simulink model "RM3_FLC"  (R2015b)
settings: Solver=ode4  StartTime=0  StopTime=200  FixedStep=0.01  MaxStep=0.01  RelTol=1e-3
values from neighbouring files (symbols this model uses):
  simu = simulationClass()    [wecSimInputFile.m]
  waves = waveClass('irregular')    [wecSimInputFile.m]
undefined symbols (not defined in the file or in its folder): body, constraint, pto
libraries: WECSim_Lib x5
settings Model: Creator=mlawson  LastModifiedBy=dforbus
settings SolverCC: ZeroCrossControl=DisableAll  AlgebraicLoopSolver=LineSearch  AutoInsertRateTranBlk=on
settings DataIOCC: LimitDataPoints=off  SaveFormat=Array  SaveOutput=off  SaveTime=off
settings OptimizationCC: SimCompilerOptimization=on
settings DebuggingCC: UnderspecifiedInitializationDetection=Classic  MergeDetectMultiDrivingBlocksExec=none  SolverPrmCheckMsg=warning  StateNameClashWarn=warning
settings HardwareCC: ProdBitPerPointer=32  ProdLargestAtomicFloat=None  ProdIntDivRoundTo=Undefined  ProdEndianess=Unspecified  ProdWordSize=32  ProdHWDeviceType=32-bit Generic
settings GRTTargetCC: GeneratePreprocessorConditionals=Disable all
settings ConfigComp: CovModelRefEnable=Off  CovSFcnEnable=off
settings SimscapeCC: SimscapeNormalizeSystem=off
settings ExplorerConfigSet: InternalSimMechanicsExplorerSettings="<ExplorerConfiguration><canonicalview>default</canonicalview><TilePanel><TileInfo><Tiles Columns=\"1\" Count=\"1\" Rows=\"1\"><Column Left=\"2\" Weight=\"1\"/><Column Left=\"1335\"/><Row Top=\"2\" Weight=\"1\"/><Row Top=\"911\"/><Tile Height=\"1\" Width=\"1\" X=\"0\" Y=\"0\"/></Tiles></TileInfo><SceneInfo><SceneViewer><BGColor><R>0.60000002384185791</R><G>0.60000002384185791</G><B>0.60000002384185791</B></BGColor><Camera><Position><X>365.37645888990272</X><Y>-369.82486814446582</Y><Z>359.64809521743916</Z></Position><Center><X>-6.7351450971904585</X><Y>2.2867358426280204</Y><Z>-12.463508769654169</Z></Center><Up><X>-0.40824829046386307</X><Y>0.40824829046386307</Y><Z>0.81649658092772615</Z></Up><Left>-57.820127362122818</Left><Right>57.820127362122818</Right><Bottom>-38.308817187253304</Bottom><Top>38.308817187253304</Top></Camera></SceneViewer></SceneInfo></TilePanel></ExplorerConfiguration>"

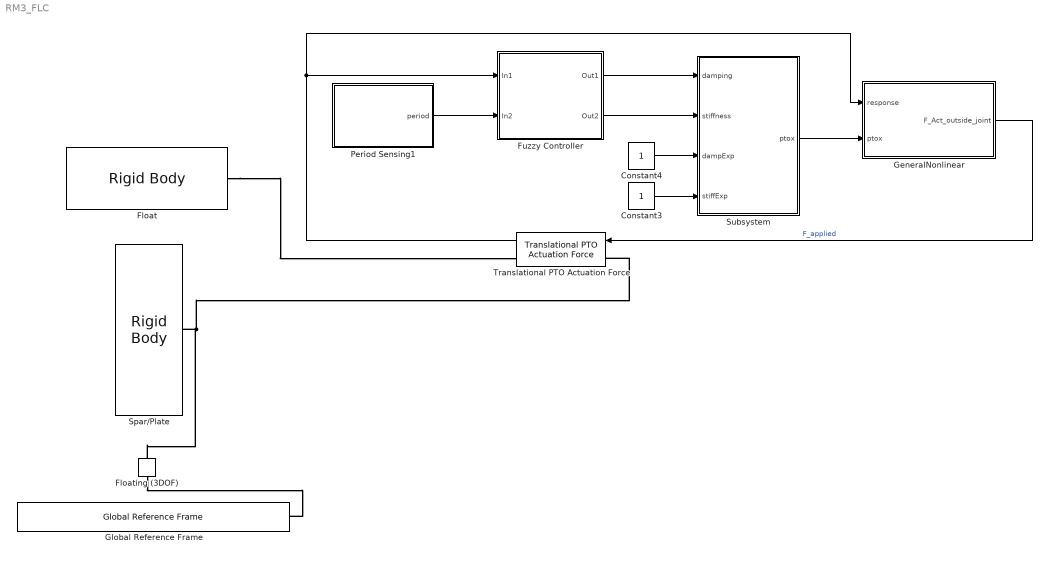
== system RM3_FLC ==
  Constant3 : Constant
  Constant4 : Constant
  Float : WECSim_Lib/Body Elements/Rigid Body  body=body(1)
      settings: AttributesFormatString=%<body>
  Floating (3DOF) : WECSim_Lib/Constraints/Floating (3DOF)  constraint=constraint(1)
      settings: AttributesFormatString=%<constraint>
  Fuzzy Controller : Subsystem
  GeneralNonlinear : Subsystem
  Global Reference Frame : WECSim_Lib/Frames/Global Reference Frame  waves=waves  simu=simu
  Period Sensing1 : Subsystem
  Spar/Plate : WECSim_Lib/Body Elements/Rigid Body  body=body(2)
      settings: AttributesFormatString=%<body>
  Subsystem : Subsystem
  Translational PTO Actuation Force : WECSim_Lib/PTOs/Translational PTO Actuation Force  pto=pto(1)
      settings: AttributesFormatString=%<pto>
  wires:
  Constant3/1 -> Subsystem/4(stiffExp)
  Subsystem/1(ptox) -> GeneralNonlinear/2(ptox)
  GeneralNonlinear/1(F_Act_outside_joint) -> Translational PTO Actuation Force/1  "F_applied"
  Constant4/1 -> Subsystem/3(dampExp)
  Translational PTO Actuation Force/1 -> GeneralNonlinear/1(response), Fuzzy Controller/1(In1)
  Fuzzy Controller/2(Out2) -> Subsystem/2(stiffness)
  Fuzzy Controller/1(Out1) -> Subsystem/1(damping)
  Period Sensing1/1(period) -> Fuzzy Controller/2(In2)
  connections:
  Floating (3DOF)/LConn1 -- Global Reference Frame/RConn1
  Spar/Plate/RConn1 -- Translational PTO Actuation Force/LConn1 -- Floating (3DOF)/RConn1
  Float/RConn1 -- Translational PTO Actuation Force/RConn1

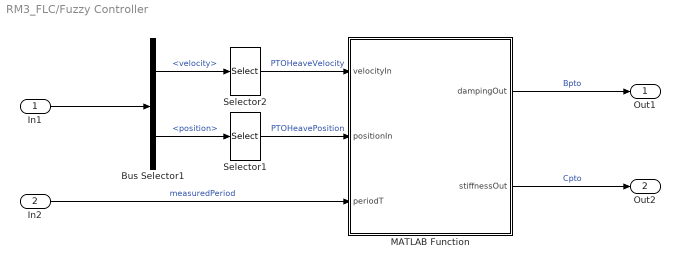
== system RM3_FLC/Fuzzy Controller ==
  In1 : Inport
  In2 : Inport  Port=2
  Bus Selector1 : BusSelector  OutputSignals=velocity,position
  MATLAB Function : MATLAB Function  TreatAsAtomicUnit=on  SystemSampleTime=0.01
  Selector1 : Selector  InputPortWidth=6  IndexOptions=Index vector (dialog)  Indices=3  OutputSizes=1
  Selector2 : Selector  InputPortWidth=6  IndexOptions=Index vector (dialog)  Indices=3  OutputSizes=1
  Out1 : Outport
  Out2 : Outport  Port=2
  wires:
  Bus Selector1/2 -> Selector1/1  "<position>"
  Selector2/1 -> MATLAB Function/1(velocityIn)  "PTOHeaveVelocity"
  Bus Selector1/1 -> Selector2/1  "<velocity>"
  In1/1 -> Bus Selector1/1
  Selector1/1 -> MATLAB Function/2(positionIn)  "PTOHeavePosition"
  MATLAB Function/1(dampingOut) -> Out1/1  "Bpto"
  MATLAB Function/2(stiffnessOut) -> Out2/1  "Cpto"
  In2/1 -> MATLAB Function/3(periodT)  "measuredPeriod"

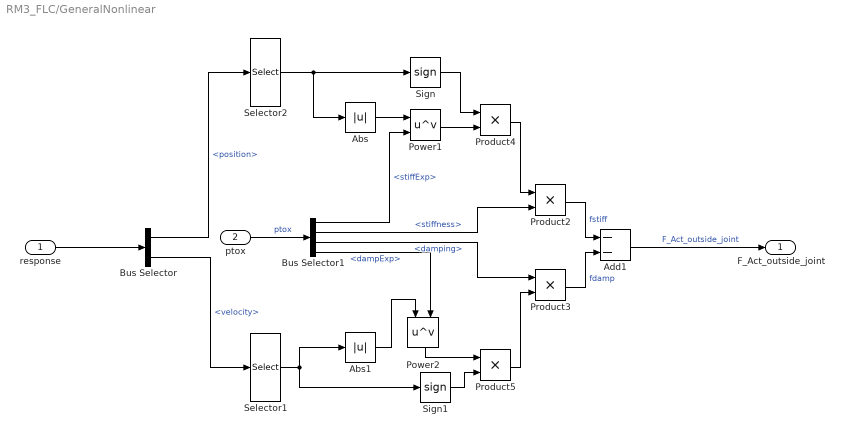
== system RM3_FLC/GeneralNonlinear ==
  response : Inport
  ptox : Inport  Port=2
  Abs : Abs
  Abs1 : Abs
  Add1 : Sum  Inputs=--
  Bus Selector : BusSelector  OutputSignals=position,velocity
  Bus Selector1 : BusSelector  OutputSignals=stiffExp,stiffness,damping,dampExp
  Power1 : Math  Operator=pow  SaturateOnIntegerOverflow=on
  Power2 : Math  Operator=pow  SaturateOnIntegerOverflow=on
  Product2 : Product  Inputs=**
  Product3 : Product  Inputs=**
  Product4 : Product
  Product5 : Product
  Selector1 : Selector  InputPortWidth=6  IndexOptions=Index vector (dialog)  Indices=3  OutputSizes=1
  Selector2 : Selector  InputPortWidth=6  IndexOptions=Index vector (dialog)  Indices=3  OutputSizes=1
  Sign : Signum
  Sign1 : Signum
  F_Act_outside_joint : Outport
  wires:
  Power2/1 -> Product5/1
  Product5/1 -> Product3/2
  Sign/1 -> Product4/1
  Bus Selector1/3 -> Product3/1  "<damping>"
  Product2/1 -> Add1/1  "fstiff"
  response/1 -> Bus Selector/1
  Bus Selector1/1 -> Power1/2  "<stiffExp>"
  Bus Selector/2 -> Selector1/1  "<velocity>"
  Selector2/1 -> Sign/1, Abs/1
  Product4/1 -> Product2/1
  Add1/1 -> F_Act_outside_joint/1  "F_Act_outside_joint"
  Abs1/1 -> Power2/1
  Product3/1 -> Add1/2  "fdamp"
  Sign1/1 -> Product5/2
  Bus Selector1/2 -> Product2/2  "<stiffness>"
  Selector1/1 -> Abs1/1, Sign1/1
  Power1/1 -> Product4/2
  Bus Selector/1 -> Selector2/1  "<position>"
  Abs/1 -> Power1/1
  ptox/1 -> Bus Selector1/1  "ptox"
  Bus Selector1/4 -> Power2/2  "<dampExp>"

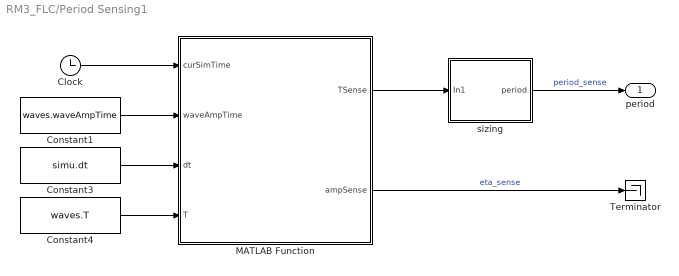
== system RM3_FLC/Period Sensing1 ==
  Clock : Clock
  Constant1 : Constant  Value=waves.waveAmpTime
  Constant3 : Constant  Value=simu.dt
  Constant4 : Constant  Value=waves.T
  MATLAB Function : MATLAB Function  TreatAsAtomicUnit=on  SystemSampleTime=0.1
  Terminator : Terminator
  sizing : Subsystem
  period : Outport
  wires:
  Constant3/1 -> MATLAB Function/3(dt)
  Constant4/1 -> MATLAB Function/4(T)
  MATLAB Function/2(ampSense) -> Terminator/1  "eta_sense"
  sizing/1(period) -> period/1  "period_sense"
  MATLAB Function/1(TSense) -> sizing/1(In1)
  Constant1/1 -> MATLAB Function/2(waveAmpTime)
  Clock/1 -> MATLAB Function/1(curSimTime)

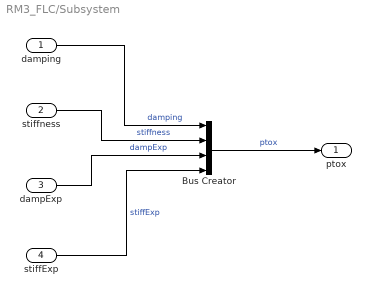
== system RM3_FLC/Subsystem ==
  damping : Inport
  stiffness : Inport  Port=2
  dampExp : Inport  Port=3
  stiffExp : Inport  Port=4
  Bus Creator : BusCreator  Inputs=4
  ptox : Outport
  wires:
  stiffness/1 -> Bus Creator/2  "stiffness"
  stiffExp/1 -> Bus Creator/4  "stiffExp"
  Bus Creator/1 -> ptox/1  "ptox"
  damping/1 -> Bus Creator/1  "damping"
  dampExp/1 -> Bus Creator/3  "dampExp"

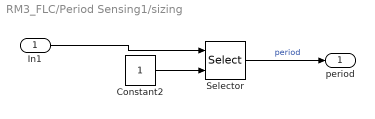
== system RM3_FLC/Period Sensing1/sizing ==
  In1 : Inport
  Constant2 : Constant
  Selector : Selector  InputPortWidth=2  IndexOptions=Index vector (port)  Indices=1  OutputSizes=1
  period : Outport
  wires:
  Constant2/1 -> Selector/2
  In1/1 -> Selector/1
  Selector/1 -> period/1  "period"

== matlab function RM3_FLC/Fuzzy Controller/MATLAB Function ==
  data: velocityIn input; positionIn input; dampingOut output; periodT input; stiffnessOut output
function [dampingOut,stiffnessOut] =...
    fuzzyLogicController(velocityIn, positionIn, periodT)
% Function to create and evaluate a fuzzy logic controller
% which implements a protection system for RM3 to limit relative movement
% between the float and spar, shedding power in the event of too-high wave conditions. The
% PTO implements an optimally linear damped control when within the travel limits,
% and applies a multiplication factor to the damping if the float is close
% to traveling out of bounds

% The functions and structures here are intended to be used as tools for the 
% general application of fuzzy logic controllers to wave energy converters.
% While not as complete as the MATLAB Fuzzy Logic Toolbox, this open source
% framework can be adapted to systems with an arbitrary number of inputs,
% outputs and rules, and can easily be expanded to include more membership
% function types, Fuzzy Operators, implication and aggregation methods, and
% defuzzification rules.

%%%%%%%%%%%%%%%%%%%%%%%%%%%%%%%%%%%%%%%%%%%%%
%% Define input membership functions (MFs) %%
%%%%%%%%%%%%%%%%%%%%%%%%%%%%%%%%%%%%%%%%%%%%%
% Input membership function (MF) structures have the following expected fields:
% type - membership function type. The following linear membership types
%           are defined 'down step' 'step' 'triangle' 'trap'
% definingPoints - the value of the input of the x axis which the linear MF
%           begins changing value e.g. a triangle starts at 0, begins climbing at the
%           first point, peaks at the second, and returns to 0 at the final.
% percentTrue - field to be occupied by the resulting value when the
%            membership function is evaluated at the system input

%%% Period Input %%%
% Min Period
period.MFs.min.type = 'down step';
begin = 3.52; finish = 5.94;
period.MFs.min.definingPoints = [begin finish];
period.MFs.min.percentTrue = NaN;

% Q1 Period
period.MFs.q1.type = 'triangle';
begin = 3.52; peak = 5.94; finish = 6.81;
period.MFs.q1.definingPoints = [begin peak finish];
period.MFs.q1.percentTrue = NaN;

% Med Period
period.MFs.med.type = 'triangle';
begin = 5.94; peak = 6.81; finish = 7.89;
period.MFs.med.definingPoints = [begin peak finish];
period.MFs.med.percentTrue = NaN;

% Q3 Period
period.MFs.q3.type = 'triangle';
begin = 6.81; peak = 7.89; finish = 12.97;
period.MFs.q3.definingPoints = [begin peak finish];
period.MFs.q3.percentTrue = NaN;

% Max Period
period.MFs.max.type = 'step';
begin = 7.89; finish = 12.97;
period.MFs.max.definingPoints = [begin finish];
period.MFs.max.percentTrue = NaN;

%%% Velocity Input %%%
% Too fast Negative Velocity Limit
velocity.MFs.fastNeg.type = 'down step';
begin = -0.50; finish = 0;
velocity.MFs.fastNeg.definingPoints = [begin finish];
velocity.MFs.fastNeg.percentTrue = NaN;

% Too Fast Positive Velocity
velocity.MFs.fastPos.type = 'step';
begin = 0; finish = 0.50;
velocity.MFs.fastPos.definingPoints = [begin finish];
velocity.MFs.fastPos.percentTrue = NaN;

%%% Position Input %%%
% Too Negative Position Limit
position.MFs.low.type = 'down step';
begin = -0.5; finish = -0.4;
position.MFs.low.definingPoints = [begin finish];
position.MFs.low.percentTrue = NaN;

% In spec position
position.MFs.middle.type = 'trap';
begin = -0.5; asc = -0.4; dec = 0.4; finish = 0.5;
position.MFs.middle.definingPoints = [begin asc dec finish];
position.MFs.middle.percentTrue = NaN;

% Too Positive Position
position.MFs.high.type = 'step';
begin = 0.4; finish = 0.5;
position.MFs.high.definingPoints = [begin finish];
position.MFs.high.percentTrue = NaN;

%%%%%%%%%%%%%%%%%%%%
%% Fuzzify Inputs %%
%%%%%%%%%%%%%%%%%%%%
% pass input values to membership functions and update struct with
% membership truth values
period.MFs = fuzzifyInputs(periodT, period.MFs);
position.MFs = fuzzifyInputs(positionIn, position.MFs);
velocity.MFs = fuzzifyInputs(velocityIn, velocity.MFs);


% organize all inputs into a single structure
inputs.period = period;
inputs.position = position;
inputs.velocity = velocity;


%%%%%%%%%%%%%%%%%%%%%%%%%%%
%% Apply Fuzzy Operators %%
%%%%%%%%%%%%%%%%%%%%%%%%%%%
% Define Rule antecedents and apply fuzzy operators to multi-input rules
% Antecedant consist of a vector of the truth values of the applicable membership 
% functions to the rule

% Rule 1 antecedent: If Period is Min
% Single input rule does not require fuzzy operator
ruleOneInputMF = [period.MFs.min.percentTrue];
ruleOneAntecedent = ruleOneInputMF;
ruleSixAntecedent = ruleOneAntecedent; % input set shared with stiffness rule 6

% Rule 2 antecedent: If Period is Q1
% Single input rule does not require fuzzy operator
ruleTwoInputMF = [period.MFs.q1.percentTrue];
ruleTwoAntecedent = ruleTwoInputMF;


% Rule 3 antecedent: If Period is median
% Single input rule does not require fuzzy operator
ruleThreeInputMF = [period.MFs.med.percentTrue];
ruleThreeAntecedent = ruleThreeInputMF;


% Rule 4 antecedent: If Period is Q3
% Single input rule does not require fuzzy operator
ruleFourInputMF = [period.MFs.q3.percentTrue];
ruleFourAntecedent = ruleFourInputMF;


% Rule 5 antecedent: If Period is Max
% Single input rule does not require fuzzy operator
ruleFiveInputMF = [period.MFs.max.percentTrue];
ruleFiveAntecedent = ruleFiveInputMF;
ruleEightAntecedent = ruleFiveAntecedent; % input set shared with stiffness rule 10

% Rule 7 antecedent: If period is q1 or med or q3
ruleSevenInputMFs = [period.MFs.q1.percentTrue period.MFs.med.percentTrue period.MFs.q3.percentTrue];
ruleSevenAntecedent = applyFuzzyOperator(ruleSevenInputMFs, 'sumOr');

% Rule 9 antecedent: If position is middle
% Single input rule does not require fuzzy operator
ruleNineInputMF = [position.MFs.middle.percentTrue];
ruleNineAntecedent = ruleNineInputMF;

% Rule 10 antecedent: If velocity is fast positive and position is high
ruleTenInputMFs = [inputs.velocity.MFs.fastPos.percentTrue  inputs.position.MFs.high.percentTrue];
ruleTenAntecedent = applyFuzzyOperator(ruleTenInputMFs, 'minAnd');

% Rule 11 antecedent: If velocity is fast negative and position is low
ruleElevenInputMFs = [inputs.velocity.MFs.fastNeg.percentTrue  position.MFs.low.percentTrue];
ruleElevenAntecedent = applyFuzzyOperator(ruleElevenInputMFs, 'minAnd');

%%%%%%%%%%%%%%%%%%%%%%%%%%%%
%% Apply Rule Implication %%
%%%%%%%%%%%%%%%%%%%%%%%%%%%%
% Specify membership functions for outputs and Generate Consequent
% Membership Functions (CMFs)

%%% Rules setting PTO Damping (Bpto) %%%

% Rule 1:  If period is min, damping is minDamping
% Base Membership Function
minPdDamping.type = 'impulse';
peak = 258893.62;
minPdDamping.definingPoints = [peak];

% Rule 2:  If period is q1, damping is q1Damping
% Base Membership Function
q1PdDamping.type = 'impulse';
peak = 858598.80;
q1PdDamping.definingPoints = [peak];

% Rule 3:  If period is med, damping is medDamping
% Base Membership Function
medPdDamping.type = 'impulse';
peak = 1353852.40;
medPdDamping.definingPoints = [peak];

% Rule 4:  If period is q3, damping is q3Damping
% Base Membership Function
q3dPdDamping.type = 'impulse';
peak = 2216704.03;
q3PdDamping.definingPoints =[peak];

% Rule 5:  If period is max, damping is maxDamping
% Base Membership Function
maxPdDamping.type = 'impulse';
peak = 35283681.68;
maxPdDamping.definingPoints = [peak];

%%% Rules setting PTO Stiffness (Cpto) %%%
%%% referred to quartiles are for the period, not the Cpto value

% Rule 6:  If period is min, Cpto is minPdStiffness
% Base Membership Function
minPdStiffness.type = 'impulse';
peak = 2480994.89;
minPdStiffness.definingPoints = [peak];

% Rule 7:  If period is q1 or med or q3, Cpto is limitStiffness
% Base Membership Function
limitStiffness.type = 'impulse';
peak = -226644.01;
limitStiffness.definingPoints = [peak];

% Rule 8: If period is max, Cpto is maxPd Stiffness
% Base Membership Function
maxPdStiffness.type = 'impulse';
peak = 14168810.64;
maxPdStiffness.definingPoints = [peak];

% Rule 9:  If position is middle damping is optimal
% Base Membership Function
optimal.type = 'triangle';
begin = -38; peak = 1; finish = 40;
optimal.definingPoints = [begin peak finish];

%%% Rules for position limiting

% Rule 10: If velocity is fast positive and position is high damping is
% overdamped

% Rule 11: If velocity is fast negative and position is low damping is
% overdamped

% Overdamped Membership Function for multiplier
overDamped.type = 'triangle';
begin = 1; peak = 40; finish = 79;
overDamped.definingPoints = [begin peak finish];

% Consequent Membership Functions for Impulse, just multiply by antecedent

% Damping
ruleOne = ruleOneAntecedent*minPdDamping.definingPoints;
ruleTwo = ruleTwoAntecedent*q1PdDamping.definingPoints;
ruleThree = ruleThreeAntecedent*medPdDamping.definingPoints;
ruleFour = ruleFourAntecedent*q3PdDamping.definingPoints;
ruleFive = ruleFiveAntecedent*maxPdDamping.definingPoints;

% Stiffness
ruleSix = ruleSixAntecedent*minPdStiffness.definingPoints;
ruleSeven = ruleSevenAntecedent*limitStiffness.definingPoints;
ruleEight = ruleEightAntecedent*maxPdStiffness.definingPoints;

%Protection
ruleNine = applyImplicationMethod(ruleNineAntecedent,optimal,'min');
ruleTen = applyImplicationMethod(ruleTenAntecedent,overDamped,'min');
ruleEleven = applyImplicationMethod(ruleElevenAntecedent,overDamped,'min');

% organize by: outputs -> fuzzy sets -> rules
% Each output struct expects a CMF field containing the fuzzy sets which
% belong to that output and a range field containing the limits of the
% output
% Each output fuzzy set struct expects a aggregation type for rules which apply
% and a rules struct containing the modified MF for those rules which apply

damping.range = [258893.62 35283681.68];

stiffness.range = [-226644.01 14168810.64];

dampingMultiplier.baseMFs.overDamped = overDamped;
dampingMultiplier.CMFs.overDamped.ruleAggregation = 'max';
dampingMultiplier.CMFs.overDamped.rules.ruleTen = ruleTen;
dampingMultiplier.CMFs.overDamped.rules.ruleEleven = ruleEleven;

dampingMultiplier.baseMFs.optimal = optimal;
dampingMultiplier.CMFs.optimal.rules.ruleNine = ruleNine;

% use NaN for no limit
dampingMultiplier.range = [1 40];

%%%%%%%%%%%%%%%%%%%%%
%% Aggregate Rules %%
%%%%%%%%%%%%%%%%%%%%%
% expected aggregation methods - 

dampRuleValues = ruleOne + ruleTwo + ruleThree + ruleFour + ruleFive;
dampTotalFirings = ruleOneAntecedent + ruleTwoAntecedent + ruleThreeAntecedent + ruleFourAntecedent + ruleFiveAntecedent;

dampingOutRaw = dampRuleValues/dampTotalFirings;


stiffRuleValues = ruleSix + ruleSeven + ruleEight;
stiffTotalFirings = ruleSixAntecedent + ruleSevenAntecedent + ruleEightAntecedent;

stiffnessOut = stiffRuleValues/stiffTotalFirings;

outputs.dampingMultiplier = dampingMultiplier;
outputs.dampingMultiplier.aggregatedFunction = aggregateCMFs(dampingMultiplier, 'max');

%%%%%%%%%%%%%%%%%%%%%%%%%%
%% Defuzzify output MFs %%
%%%%%%%%%%%%%%%%%%%%%%%%%%
% Defuzzify final output membership functions and assign crisp values
% expected defuzzification methods: centroid, bisector, mean of maxima (MOM),
% largest of maxima (LOM), smallest of maxima (SOM)

 if ~(ruleNineAntecedent) && ~(ruleTenAntecedent) && ~(ruleElevenAntecedent)
    dampingFactor = 1; %default if no rules fires
 else
    dampingFactor = defuzzify(outputs.dampingMultiplier, 'bisector');
    if dampingFactor > 1
        dampingFactor = 1; % overdamp only
    end
 end
 
 dampingOutIntermediate = dampingOutRaw*dampingFactor;
 
 dampingOut = dampingOutIntermediate(1);

end
%%%%%%%%%%%%%%%%%%
%% End of Main %%
%%%%%%%%%%%%%%%%%%
% begin supporting functions

function fuzzufiedInput = fuzzifyInputs(inValue, MFs)
% Function to fuzzify crisp input variables
% inputs: 
%   invalue - crisp input value
%   MFs - struct of fuzzy set membership functions for an input
% outputs: 
%   fuzzufiedInput - updated MFs struct with fuzzy truth value for each MF

    % list of memberships for this input
    listMFs = fieldnames(MFs);

    % go through each membership function
    for k=1:numel(listMFs)
        thisMF = MFs.(listMFs{k});

        mfType = thisMF.type;

        %calculate its percentTrue strength based on type
        switch mfType
            case 'triangle'
                MFs.(listMFs{k}).percentTrue = tri_MF(inValue,...
                    MFs.(listMFs{k}).definingPoints(1), MFs.(listMFs{k}).definingPoints(2), MFs.(listMFs{k}).definingPoints(3), 1);
            case 'step'
                MFs.(listMFs{k}).percentTrue = open_trap_right(inValue,...
                     MFs.(listMFs{k}).definingPoints(1), MFs.(listMFs{k}).definingPoints(2), 1);
            case 'down step'
                 MFs.(listMFs{k}).percentTrue = open_trap_left(inValue,...
                     MFs.(listMFs{k}).definingPoints(1), MFs.(listMFs{k}).definingPoints(2), 1);
            case 'trap'
                 MFs.(listMFs{k}).percentTrue = trap(inValue,...
                     MFs.(listMFs{k}).definingPoints(1), MFs.(listMFs{k}).definingPoints(2), MFs.(listMFs{k}).definingPoints(3), MFs.(listMFs{k}).definingPoints(4), 1);
            otherwise
                disp('membership function type not defined');
        end
    end

    fuzzufiedInput = MFs;

end

function membership = tri_MF(inValue, begin, peak, finish, maxTruth)
% Evaluate input according to triangular MF
% inputs: 
%   inValue - system input value 
%   begin - input value triangle begins to rise, before which truth value is 0
%   peak - input value triangle peaks and begins to fall
%   finish - input value triangle returns to 0, after which which truth value is 0
%   maxTruth - truth value for peak input, default 1 for input MFs
% outputs:
%   membership - truth value between 0 and 1 corresponding to the input    
%
    if inValue < peak
        if inValue <= begin
            membership = 0;
        else
            membership = (maxTruth/(peak - begin)) * (inValue-peak) + maxTruth;
        end
    elseif inValue > peak
        if inValue >= finish
            membership = 0;
        else
            membership = ((-1*maxTruth)/(finish - peak)) * (inValue-peak) + maxTruth;
        end
    else
        membership = maxTruth;
    end
end

function membership = open_trap_left(inValue, begin, finish, maxTruth)
% Evaluate input according to falling step membership function
% inputs: 
%   inValue - system input value 
%   begin - input value step begins to fall, before which truth value is 1
%   finish - input value trap reaches 0, after which which truth value is 0
%   maxTruth - truth value for input below 'begin', default 1 for input MFs
% outputs:
%   membership - truth value between 0 and 1 corresponding to the input    
%
    if inValue < begin
        membership = maxTruth;
    elseif inValue > finish
        membership = 0;
    else
        membership = (maxTruth/(begin - finish))*(inValue - begin) + maxTruth;
    end
end

function membership = open_trap_right(inValue, begin, finish, maxTruth)
% Evaluate input according to rising step membership function
% inputs: 
%   inValue - system input value 
%   begin - input value step begins to rise, before which truth value is 0
%   finish - input value trap reaches 1, after which which truth value is 1
%   maxTruth - truth value for input above 'finish', default 1 for input MFs
% outputs:
%   membership - truth value between 0 and 1 corresponding to the input   

    if inValue < begin
        membership = 0;
    elseif inValue > finish
        membership = maxTruth;
    else
        membership = (maxTruth/(finish - begin))*(inValue - finish) + maxTruth;
    end
end

function membership = trap(inValue, begin, asc, dec, finish, maxTruth)
% Evaluate input according to trapezoidal MF
% inputs: 
%   inValue - system input value 
%   begin - input value at which trapezoid begins to rise, before which truth value is 0
%   asc - input value at which trapezoid reaches plateau value
%   dec - input value at which trapezoid returns to 0, after which truth value is 0
%   maxTruth - truth value for plateau inputs, default 1 for input MFs
% outputs:
%   membership - truth value between 0 and 1 corresponding to the input    
%
    if ( inValue < begin ) || ( inValue > finish )
        membership = 0;
    elseif inValue < asc
        membership = (maxTruth/(asc-begin))*(inValue - begin);
    elseif inValue > dec
        membership = (maxTruth/(dec-finish))*(inValue - finish);
    else
        membership = maxTruth;
    end
end


function antecedentTruth = applyFuzzyOperator(inputMembershipTruth, fuzzyOperator)
% applies a fuzzy operator to produce a single 
% antecedent value for multi-input fuzzy rules
% Inputs: 
%       inputMembershipTruth - vector of analog truth values for
%       input membership function values relevant to rule
%       fuzzyOperator - Fuzzy operator to select a single truth value for the
%       antecedent of the rule
    switch fuzzyOperator
        case 'minAnd'
            antecedentTruth = min(inputMembershipTruth);
        case 'prodAnd'
            antecedentTruth = prod(inputMembershipTruth);
        case 'sumOr'
            antecedentTruth = sum(inputMembershipTruth);
        case 'maxOr'
            antecedentTruth = max(inputMembershipTruth);
        case 'average'
            antecedentTruth = mean(inputMembershipTruth);
        otherwise
            disp('Specified Fuzzy Operator is not defined');
    end
end

function consequentMF = applyImplicationMethod(antecedent, outputMembership, implicationMethod)
% function to implicate rules
% inputs:
%   antecedent - single truth value for the rule's antecedent
%   outputMembership - membership funciton structure for output
%   implicationMethod - an implication method
% outputs: 
%   consequentMF - membership function shaped by the antecedent
    if (antecedent == 1) || (antecedent == 0) || strcmp(implicationMethod,'prod')
        outCopy = outputMembership;
        outCopy.maxVal = antecedent;
        consequentMF = outCopy;
    elseif strcmp(implicationMethod,'min')
        switch outputMembership.type
            case 'trap'
                outTrap = outputMembership;
                outTrap.maxVal = antecedent;
                outTrap.definingPoints(2) = antecedent * (outputMembership.definingPoints(2) - outputMembership.definingPoints(1)) + outputMembership.definingPoints(1);
                outTrap.definingPoints(3) = antecedent * (outputMembership.definingPoints(3) - outputMembership.definingPoints(4)) + outputMembership.definingPoints(4);
                consequentMF = outTrap;
            case 'step'
                outStep = outputMembership;
                outStep.maxVal = antecedent;
                outStep.definingPoints(2) = antecedent * (outputMembership.definingPoints(2) - outputMembership.definingPoints(1)) + outputMembership.definingPoints(1);
                consequentMF = outStep;
            case 'down step'
                outDownStep = outputMembership;
                outDownStep.definingPoints(1) = antecedent * (outputMembership.definingPoints(1) - outputMembership.definingPoints(2)) + outputMembership.definingPoints(2);
                outDownStep.maxVal = antecedent;
                consequentMF = outDownStep;
            case 'triangle' % Chop the top off
                outTri.type = 'trap';
                outTri.definingPoints = zeros(1,4);
                outTri.definingPoints(1) = outputMembership.definingPoints(1);
                outTri.definingPoints(4) = outputMembership.definingPoints(3);
                outTri.definingPoints(2) = antecedent * (outputMembership.definingPoints(2) - outputMembership.definingPoints(1)) + outputMembership.definingPoints(1);
                outTri.definingPoints(3) = antecedent * (outputMembership.definingPoints(2) - outputMembership.definingPoints(3)) + outputMembership.definingPoints(3);
                outTri.maxVal = antecedent;
                consequentMF = outTri;
            otherwise
                disp('membership function specified for output not defined');
        end
    else
        disp('Specified implication method is not defined');
        consequentMF = 0;
    end
end

function mfTruth = evalMF(inValue, MF)
% General function to evaluate membership functions may not have a max of 1
% inputs:
%   inValue - value to evaluate membership for
%   MF - membership function struct which expects a maxVal field
% outputs:
%   single truth value
%

mfType = MF.type;
        %calculate its percentTrue strength based on
        switch mfType
            case 'triangle'
                mfTruth = tri_MF(inValue,...
                    MF.definingPoints(1), MF.definingPoints(2), MF.definingPoints(3),  MF.maxVal);
            case 'step'
                mfTruth = open_trap_right(inValue,...
                     MF.definingPoints(1), MF.definingPoints(2), MF.maxVal);
            case 'down step'
                 mfTruth = open_trap_left(inValue,...
                     MF.definingPoints(1), MF.definingPoints(2), MF.maxVal);
            case 'trap'
                 mfTruth = trap(inValue,...
                     MF.definingPoints(1), MF.definingPoints(2), MF.definingPoints(3), MF.definingPoints(4), MF.maxVal);
            otherwise
                mfTruth = NaN;
                disp('membership function type not defined');
        end
end

function singleTruthFunction = performAgg(truthMatrix, aggregationMethod)
% function to aggreate rules
% inputs:
%   truthMatrix: matrix where each row represents the truth value of the
%   corresponding rule's membership function, evaluated at the necessary
%   points to get a complete detailed aggregation
%

    switch aggregationMethod
        case 'max'
            singleTruthFunction = max(truthMatrix,[],1);
        case 'min'
            singleTruthFunction = min(truthMatrix,[],1);
        case 'mean'
            singleTruthFunction = mean(truthMatrix,[],1);
        case 'prod'
            singleTruthFunction = truthMatrix(1,:)
            for r = 2:length(truthMatrix(:,1))
                singleTruthFunction = truthMatrix(r,:).*singleTruthFunction;
            end
        case 'sum'
            singleTruthFunction = truthMatrix(1,:);
            if length(truthMatrix(:,1)) > 1
                for r = 2:length(truthMatrix(:,1))
                    singleTruthFunction = truthMatrix(r,:) + singleTruthFunction;
                end
            end
        otherwise
            disp('specified aggregation method not defined');
    end
end

function aggregatedMF = aggregateCMFs(outputName, aggregationMethod)
% function to aggregate all rules' MFs which apply to an output fuzzy set,
% then to aggregate all sets which apply to the output
% inputs: 
%   outputName - structure containing the fuzzy sets for each input, and
%   consequent membership functions for each rule of each set
%   aggregationMethod - an aggregation method for the sets
% outputs:
%   aggregatedMF - 2 row vector representing the final aggregated membership 
%   function for the output with the first row being the output values (x
%   axis) and the second row as the corresponding truth value (y axis)

listStates = fieldnames(outputName.CMFs);
outMin = outputName.range(1);
outMax = outputName.range(2);

% Loop 1 to aggregate rules for each state/MF (e.g. rule 2 and 3 both affect
% overdamped set, their consequent MF must be combined)
for p=1:numel(listStates)
    thisCMF = outputName.CMFs.(listStates{p});
    
    listRules = fieldnames(thisCMF.rules);
    if numel(listRules) > 1
        if (thisCMF.ruleAggregation)
            ruleAgg = thisCMF.ruleAggregation;
        else
            disp('If multiple rules affect a member function a rule aggregation must be specified');
        end
    end
    
    % get unique list of defining points for this state (from all rules for
    % this state)

    % first loop to get the length of all defining points for this state for
    % preallocation purposes
    ruleRangeMaxLength = 0;
    for s=1:numel(listRules)
        thesePoints = outputName.CMFs.(listStates{p}).rules.(listRules{s}).definingPoints;
        ruleRangeMaxLength = ruleRangeMaxLength + numel(thesePoints);
    end
    
    %Now assign all points to range vector
    fullRuleRange = NaN(1,ruleRangeMaxLength);
    fullRuleRangeIndex=1;
    for s=1:numel(listRules)
        thesePoints = outputName.CMFs.(listStates{p}).rules.(listRules{s}).definingPoints;
        for t = 1:numel(thesePoints)
            fullRuleRange(fullRuleRangeIndex) = thesePoints(t);
            fullRuleRangeIndex = fullRuleRangeIndex+1;
        end
        
    end
    
    % remove duplicates
    uniqueRuleRange = unique(fullRuleRange(~isnan(fullRuleRange)));

    
    % loop through comparing each rule and add any rule intersections to
    % the list of defining points
    
    % first count the max number of points the intersections could add, for
    % allocation purposes
    ruleIntersectionsMaxLength = 0;
    for s=1:numel(listRules)
        compareRuleOne = thisCMF.rules.(listRules{s});
        
        for t = (s+1):numel(listRules)
            compareRuleTwo = thisCMF.rules.(listRules{t});
            
            ruleOneTruth = NaN(1,numel(uniqueRuleRange));
            ruleTwoTruth = NaN(1,numel(uniqueRuleRange));
            
            % create y values for each rule MF
            for m = 1:numel(uniqueRuleRange)
               uniqueRuleRange(m);
               ruleOneTruth(m) = evalMF(uniqueRuleRange(m),compareRuleOne);
               ruleTwoTruth(m) = evalMF(uniqueRuleRange(m),compareRuleTwo);
            end
            
            ruleX = MFintersect(uniqueRuleRange, ruleOneTruth, ruleTwoTruth);
            ruleIntersectionsMaxLength = ruleIntersectionsMaxLength + numel(ruleX);
        end
    end
    
    % preallocate
    rangeWithIntersections = NaN(1,ruleIntersectionsMaxLength);
    
    % Now go through and assign
    intersectionIndex = 1;
    for s=1:numel(listRules)
        compareRuleOne = thisCMF.rules.(listRules{s});
        
        for t = (s+1):numel(listRules)
            compareRuleTwo = thisCMF.rules.(listRules{t});
            
            ruleOneTruth = NaN(1,numel(uniqueRuleRange));
            ruleTwoTruth = NaN(1,numel(uniqueRuleRange));
            
            % create y values for each rule MF
            for m = 1:numel(uniqueRuleRange)
               uniqueRuleRange(m);
               ruleOneTruth(m) = evalMF(uniqueRuleRange(m),compareRuleOne);
               ruleTwoTruth(m) = evalMF(uniqueRuleRange(m),compareRuleTwo);
            end
            
            ruleX = MFintersect(uniqueRuleRange, ruleOneTruth, ruleTwoTruth);
            ruleIntersections = ruleX;
            for n = 1:numel(ruleIntersections(1,:))
                rangeWithIntersections(intersectionIndex) = ruleIntersections(1,n);
                intersectionIndex = intersectionIndex + 1;
            end
        end
    end
    
    % remove duplicates
    %rangeWithIntersections
    %uniqueRangeIntersections = unique(rangeWithIntersections);
    
    % combine the two and remove any lingering NaN
    finalOutRange = [rangeWithIntersections  uniqueRuleRange];
    uniqueFinalRange = unique(finalOutRange(~isnan(finalOutRange)));
 
    % Now we have the list of output values which define the corners and
    % possible intersections of all rules for this MF state. Define a
    % matrix where each row will be a rule MF for aggregation for all
    % points along the relevant range
    
    stateRulesMat = zeros(numel(listRules),numel(uniqueFinalRange));
    
    for row=1:numel(listRules)
        thisRule = thisCMF.rules.(listRules{row});
        for col = 1:numel(uniqueFinalRange)
            stateRulesMat(row,col) = evalMF(uniqueFinalRange(col),thisRule);
        end
    end
    
    % Finally can aggregate rules without losing any MF resolution
    outVari.(listStates{p}).func = [uniqueFinalRange; performAgg(stateRulesMat, aggregationMethod)];
        
end

% Now aggregate all the set MFs (e.g. overdamped and optimal)


stateList = fieldnames(outVari);

% this loop get all the X over each state MF
% first loop that counts for preallocate
maxDefiningPointsCount = 0;
for p = 1:numel(stateList)
    thisState = outVari.(stateList{p});
    maxDefiningPointsCount = maxDefiningPointsCount + numel(thisState.func(1,:));
end

% preallocate
outRange = NaN(1,maxDefiningPointsCount);
outRangeIndex = 1;

% second loop assigns
for p = 1:numel(stateList)
    thisState = outVari.(stateList{p});

    for q = 1:numel(thisState.func(1,:))
        outRange(outRangeIndex) = thisState.func(1,q);
        outRangeIndex = outRangeIndex + 1;
    end
    
end

outRangeLimits = [outRange outMin outMax];


uniqueOutRange = unique(outRangeLimits);

stateOutMat = zeros(numel(stateList),numel(uniqueOutRange));
for row = 1:numel(stateList)
    thisFuncX = outVari.(stateList{row}).func(1,:);
    thisFuncT = outVari.(stateList{row}).func(2,:);
    for col = 1:numel(uniqueOutRange)
        if (uniqueOutRange(col) > max(thisFuncX)) || (uniqueOutRange(col) < min(thisFuncX))
            stateOutMat(row,col) = interp1(thisFuncX,thisFuncT,uniqueOutRange(col),'nearest','extrap');
        else
            stateOutMat(row,col) = interp1(thisFuncX,thisFuncT,uniqueOutRange(col),'linear');
        end
    end
end

% loop through rows of stateOutMat vs unique out range to count intersections
maxSetIntersects = 0;
[numSetRows ~] = size(stateOutMat);
for s = 1:numSetRows
    setCompareOne = stateOutMat(s,:);
    
    for t = s+1:numSetRows
        setCompareTwo = stateOutMat(t,:);
        
        setX = MFintersect(uniqueOutRange, setCompareOne, setCompareTwo);
        maxSetIntersects = maxSetIntersects + numel(setX);
        
    end
end

% preallocate
setIntersectionX = NaN(1,maxSetIntersects);
intersectionCount = 1;

% loop to assign them
for s = 1:numSetRows
    setCompareOne = stateOutMat(s,:);
    
    for t = s+1:numSetRows
        setCompareTwo = stateOutMat(t,:);
        
        setX = MFintersect(uniqueOutRange, setCompareOne, setCompareTwo);
        
        for u = 1:numel(setX(1,:))
            setIntersectionX(intersectionCount) = setX(1,u);
            intersectionCount = intersectionCount + 1;
        end
        
    end
end

% add them to range
finalOutRangeWithIntersects = [uniqueOutRange setIntersectionX];
% removeNaNs and dups
finalRange = unique(finalOutRangeWithIntersects(~isnan(finalOutRangeWithIntersects)));

% re-create state out mat with new output range
finalStateOutMat = NaN(numel(stateList),numel(finalRange));
for row = 1:numel(stateList)
    thisFuncX = uniqueOutRange;
    thisFuncT = stateOutMat(row,:);
    
    for col = 1:numel(finalRange)
        if (finalRange(col) > max(thisFuncX)) || (finalRange(col) < min(thisFuncX))
            finalStateOutMat(row,col) = interp1(thisFuncX,thisFuncT,finalRange(col),'nearest','extrap');
        else
            finalStateOutMat(row,col) = interp1(thisFuncX,thisFuncT,finalRange(col),'linear');
        end
    end
end



%Finally, finally, finally can aggregate all output's set MFs without losing resolution
aggregatedFunction = performAgg(finalStateOutMat, aggregationMethod);

% return as a linear interpolate function
aggregatedMF = [finalRange; aggregatedFunction];

 end

function crisp = defuzzify(outputFun, defuzzificationMethod)
% function to call relevant defuzzification function

outMin = outputFun.range(1);
outMax = outputFun.range(2);

func = outputFun.aggregatedFunction;
switch defuzzificationMethod
    case 'centroid'
        crisp = getCentroidX(func);
    case 'bisector'
        crisp = bisectSearch(func,min(func(1,:)),max(func(1,:)));
    case 'LOM'
        crisp = maxima(func,'largest');
    case 'MOM'
        crisp = maxima(func,'mean');
    case 'SOM'
        crisp = maxima(func,'smallest');
    otherwise disp('Specified defuzzification method not defined');
        crisp = NaN;
end

% Keep it in range
if crisp(1) > outMax && ~isnan(outMax)
    crisp = outMax;
elseif crisp(1) < outMin  && ~isnan(outMin)
    crisp = outMin;
end

end

function centroX = getCentroidX(curve)
% function to return output value corresponding to MF centroid

    if curve(2,end) ~= 0
        polydCurve = [curve [curve(1, end) ; 0 ] ];
    else
         polydCurve = curve;
    end

    polyin = polyshape(polydCurve','Simplify',true);
    polyin = simplify(polyin,'KeepCollinearPoints',false);
    [x,~] = centroid(polyin);    
    centroX = x;
end

function xBisect = bisectSearch(curve,searchMin,seaarchMax)
% function to return output value corresponding to MF bisector

    xBisect = 0;
    fullX = curve(1,:);
    fullY = curve(2,:);

    totalArea = trapz(fullX,fullY);
    
    midX = (searchMin + seaarchMax)/2;
    midY = interp1(fullX,fullY,midX,'linear');
    
    
    halfXTest = [fullX(fullX < midX) midX];
    halfYTestLen = numel(fullX(fullX < midX));
    halfYTest = [fullY(1:halfYTestLen) midY];
    halfAreaTest = trapz(halfXTest,halfYTest);
    
    if round(halfAreaTest) == round(0.5*totalArea)
        xBisect = midX;
    elseif halfAreaTest > 0.5*totalArea
        xBisect = bisectSearch(curve,searchMin,midX);
    elseif halfAreaTest < 0.5*totalArea
        xBisect = bisectSearch(curve,midX,seaarchMax);
    end
end

function aMax = maxima(curve,type)
% function to return output value corresponding to MF maxima type

aMax = 0;
fullX = curve(1,:);
fullY = curve(2,:);

% if there is a single most true point
if size(fullY(fullY == max(fullY))) == 1
    % return the x
    aMax = fullX(find(fullY==max(fullY)));
else
    switch type
        case 'largest'
            % largest = highest absolute value 
            maximaXs = fullX(find(fullY==max(fullY)));
            maximaXsMag = abs(maximaXs);
            
            if size(maximaXsMag(maximaXsMag == max(maximaXsMag))) == 1
                % if there's only 1 max abs value, return the x
                aMax = maximaXs(find(maximaXsMag==max(maximaXsMag)));
            else
                % if there's a tie (i.e. the corresponding positive and
                % negative x are both the most true) return the negative
                % one
                aMax = maximaXs(find(maximaXs==-1*max(maximaXsMag)));
            end
        case 'mean'
            maximaXs = fullX(find(fullY==max(fullY)));
            aMax = (max(maximaXs) + min(maximaXs))/2;
        case 'smallest'
            % smallest = lowest absolute value 
            maximaXs = fullX(find(fullY==max(fullY)));
            maximaXsMag = abs(maximaXs);
            
            if size(maximaXsMag(maximaXsMag == min(maximaXsMag))) == 1
                % if there's only 1, return the x
                aMax = maximaXs(find(maximaXsMag==min(maximaXsMag)));
            else
                % if there's a tie (i.e. the corresponding positive and
                % negative x are both the most true values) return the 
                % negative one
                aMax = maximaXs(find(maximaXs==-1*min(maximaXsMag)));
            end
    end

end

end

function intersectionsX = MFintersect(X, Y1, Y2)

% get two consecutive sets of truth values. subtract them from each other,
% and compare the signs. if they're different, find the interesection

% if it does, solve the 2 linear equations for the intersection.

% count for pre-allocate
intersectionsCount = 0;
for i = 2:numel(X)
    if (sign(Y1(i-1)-Y2(i-1)) ~= sign(Y1(i)-Y2(i)))
        intersectionsCount = intersectionsCount + 1;
    end
end

% preallocate
intersectionsX = NaN(1,intersectionsCount);
intersectionNumber = 1;
    
for i = 2:numel(X)

    % check if who's on top changed
    if (sign(Y1(i-1)-Y2(i-1)) ~= sign(Y1(i)-Y2(i)))
        
        % line slopes in intersection interval
        M1 = (Y1(i-1)-Y1(i))/(X(i-1)-X(i));
        M2 = (Y2(i-1)-Y2(i))/(X(i-1)-X(i));
        
        % X value of intersection
        intersectionsX(intersectionNumber) = ...%find the x value of intersections
            X(i) + (Y2(i)-Y1(i))/(M1-M2);
        intersectionNumber = intersectionNumber + 1;
    end
    
    if intersectionNumber > intersectionsCount
        break;
    end
end    


end

== matlab function RM3_FLC/Period Sensing1/MATLAB Function ==
  data: curSimTime input; TSense output size=[1 2]; waveAmpTime input; dt input; ampSense output; T input
function [TSense,ampSense] = getPeriod(curSimTime, waveAmpTime, dt, T)

% This function sort of pretends we don't know the full time series for
% wave amplitude since for control purposes, we won't. Use a rolling sample
% window of the wave height and DFT to get an approximate period for
% input into the controller. This way the control can respond to a more
% "instantaneous" value for period. In some instances we may need to
% "cheat" and access Waves.T, or the entire series, in order to pick a
% default value. A more realistic / suitable default value might be
% a known average period for a given location / season / time of day.

% REQUIREMENTS: - a fixed step simulation (simu.solver = 'ode4'; simu.dt is defined)
% does not support etaImport waveclass (just need to pick a default value instead of Waves.T)

% Inputs: 
% curSimTime: the current simulation time
% waveAmpTime: the wave aplitude timeseries
% dt: simulation step
% T: default wave period

% Outputs
% Tsense: approximate period
% ampSense: current amplitude value


if curSimTime == 0 % no history...
    TSense = T;
    ampSense = 0;
else
    
    t = waveAmpTime(:,1);
    amp = waveAmpTime(:,2);

    % Time series of amplitudes from simulation start to current time step
    allPastt = t(t <= curSimTime);
    allPastSamples = numel(allPastt);
    allPastAmp = amp(1:allPastSamples);
    
    % Current Amplitude
    ampSense = allPastAmp(end);

    % Create a 5-ish cycle sample window
    samplesPerCycle = T/dt;
    if curSimTime < 5*T
        windowSamples = allPastSamples; % use what we got
    else
        windowSamples = 5*samplesPerCycle;
    end

    windowPastt = allPastt(end-windowSamples+1:end);
    windowPastAmp = allPastAmp(end-windowSamples+1:end);

    % Sampling frequency
    fs = 1/dt;

    %Signal Length
    L = windowSamples;

    % Calculate fft
    ampDftMags = abs(fft(windowPastAmp));

    %%Single-sided magnitude spectrum with frequency axis in Hertz
    % Each bin frequency is separated by fs/L Hertz.
    binVals = [0 : L-1];
    fHz = binVals*fs/L;
    L_2 = ceil(L/2);

    freqs = fHz(1:L_2);
    mags = ampDftMags(1:L_2);

    [~, dPd] = max(mags);
    TSense = 1/freqs(dPd);


    if TSense == Inf
       TSense = T;
    end
end
end
